simulink model "finalcode"  (R2020a)
settings: Solver=FixedStepDiscrete  StartTime=0.0  StopTime=1  FixedStep=0.0005  RelTol=1e-3  EnableMultiTasking=on
undefined symbols (not defined in the file): acc_calmax1, acc_calmax2, acc_calmin1, acc_calmin2, akemancanshu, angle_middle, bre, bre_calmax, bre_calmin, chasuniujvvvv_hou, chasuniujvvvv_qian, chasuuuu, ecucoder_acal, I_AN01_5K1, I_AN03_5V, I_AN04_5V, kd, kddd, ki, kiii, kp, kppp, leftmax, O_SW06_HS1A, P11111, P22222, PIDmodel, PPPP, rightmax, slip, slip_big, slip_little, slipmodel, T_add, T_del, tiaoshi, TTTTTyouren, vvvv, zhiling
libraries: ec5744lib x305, canmsglib x97, simulink x23
(part 9 of 11)

== matlab function finalcode/转向自动标定/转向自动标定/Subsystem/MATLAB Function ==
  data: steer output; y output; rm input; lm input; bianmaqi input; k output; d output
function [steer,y,k,d] = fcn(rm,lm,bianmaqi)
%使用前请将转向打到最左侧
lm=lm+3000;
rm=rm-3000;
k=0;
d=0;
  persistent i  A B;
     % 初始化状态变量
    if isempty(i)
        i = 0;
        A=zeros(120,1);
        B=zeros(120,1);
    end
 
    if i>20&&i<=140  
        j=i-20;
        delta=(rm-lm)/120;
        steer= lm+j*delta ;
        if (j>=1&&j<=120)
            B(j,1)=steer-delta;
            A(j,1)=bianmaqi;
        end
        
    else
      if i>=140
            N=length(A);
%             bb=0;
%             aa=0;
%             for l=1:120
%                 bbb=bb+B(l,1);
%                 aaa=aa+A(l,1);
%             end
%             bbar=bbb/120;
%             abar=aaa/120;
            k=(sum(B.*A)-N*mean(B)*mean(A))/(sum(A.^2)-N*mean(A)^2);
            d=mean(B)-k*mean(A);
%             steer=single(d);
        end
        steer=lm;
    end

    i=i+1;
  persistent time  a b;
     % 初始化状态变量
    if isempty(time)
        time = 0;
   
        a=5;
        b=10;
    end
    if mod(abs(time), 2) == 0
        result = 1;
    else
        result = 0;
    end
    if time<b&&result==0
    y=6;
 
    elseif time<b&&result==1
    y=15;
  
    elseif time>=b
        if result==1
            y=79;
        else
            y=63;
        end
    else
        y=6;
    end   
    time=time+1;
 
%     
%       persistent time1;
%      % 初始化状态变量
%     if isempty(time1)
%         time1 = 0;
%     end
%     if mod(time1, 2) == 0
%         result1 = 1;
%     else
%         result1 = 0;
%     end
%     if time1<2
%     y=6;
%  
%     elseif time1>=2&&time1<4
%     y=15;
%   
%     elseif time1>=4
%         if result1==1
%             y=79;
%         else
%             y=63;
%         end
%     else
%         y=6;
%     end   
%     time1=time1+1;
   
end

== matlab function finalcode/Subsystem/run/analog_input/有人/踏板标定/踏板冲突 ==
  data: acc_fin_sig1 input; y output; acc_fin_sig2 input; bre_ori_sig input; bre input
function y = fcn(acc_fin_sig1,  acc_fin_sig2,bre_ori_sig,bre)
if (acc_fin_sig1>0.3&&bre_ori_sig+bre>=1)||bre_ori_sig+bre>=2
    y=0;
elseif (acc_fin_sig1==0||acc_fin_sig2==0)
    y=0;
else
    y=acc_fin_sig2;
end

== matlab function finalcode/Subsystem/run/analog_input/有人/踏板标定/Subsystem1/MATLAB Function ==
  data: u input; y output
function y = fcn(u)
if u==0
    y=0;
else
    y=1;
end

== matlab function finalcode/Subsystem/run/analog_input/有人/Subsystem1/MATLAB Function ==
  data: v input; T output
function T = fcn(v)
%#codegen
if v<6000*1.88e-3
    T=2100;
elseif v>11000*1.88e-3
    T=800;
else
    T=1100;
end

== matlab function finalcode/Subsystem/run/analog_input/有人/Subsystem1/MATLAB Function1 ==
  data: T input; TP output
function TP= fcn(T)
if T<10
    TP=0;
else
    TP=T;
end

== matlab function finalcode/Subsystem/run/ctrl/Subsystem1/control_strategy/E,H ==
  data: A input; E output; B input; Q input; R input; F input; N input; H output; J output
function [E,H,J] = MPC_Matrices(A,B,Q,R,F,N)
    n=size(A,1); % A是n*n矩阵,得到n
    p=size(B,2); % B是n*p矩阵,得到p
    M=[eye(n);zeros(N*n,n)]; % 初始化M矩阵,M矩阵是(N+1)n*n的,
                             % 它上面是n*n个"I",这一步先把下半部分写成0
    C=zeros((N+1)*n,N*p); % 初始化C矩阵,这一步令它有(N+1)n*NP个0
     D=zeros(1,N*p);
    % 定义M和C
    tmp=eye(n); % 定义一个n*n 的 I 矩阵
    % 更新Ｍ和C
    for i=1:N % 循环,i从1到N
        rows =i*n+(1:n); %定义当前行数,从i*n开始，共n行
        C(rows,:)=[tmp*B,C(rows-n, 1:end-p)]; %将c矩阵填满
        tmp= A*tmp; %每一次将tmp左乘一次A
        M(rows,:)=tmp; %将M矩阵写满
    end
    % 定义Q_bar和R_bar
    Q_bar = kron(eye(N),Q);
    Q_bar = blkdiag(Q_bar,F);
    R_bar = kron(eye(N),R);
    % 计算G,E,H
    G=M'*Q_bar*M; % G: n*n
    E=C'*Q_bar*M; % E: NP*n
    H=C'*Q_bar*C+R_bar; % NP*NP
for i=1:N % 循环,i从1到N
     D(i)= 0.17;
end
  J=C'*Q_bar*D'

== matlab function finalcode/Subsystem/run/ctrl/Subsystem1/control_strategy/MATLAB Function ==
  data: slip_ratio_fl input; torque_cmd_fl output; slip_ratio_fr input; slip_ratio_rl input; slip_ratio_rr input; desired_slip_ratio input; driver_torque_cmd_fl input; driver_torque_cmd_fr input; driver_torque_cmd_rl input; driver_torque_cmd_rr input; dt input; B input; C input; D input; E input; wheel_radius input; torque_cmd_fr output; torque_cmd_rl output; torque_cmd_rr output
function [torque_cmd_fl, torque_cmd_fr, torque_cmd_rl, torque_cmd_rr] = SlipRatioControlWithMagicFormula(slip_ratio_fl, slip_ratio_fr, slip_ratio_rl, slip_ratio_rr, desired_slip_ratio, driver_torque_cmd_fl, driver_torque_cmd_fr, driver_torque_cmd_rl, driver_torque_cmd_rr, dt, B, C, D, E, wheel_radius)

    % 定义持久变量来存储每个轮胎的上一次误差
    persistent e_prev_fl e_prev_fr e_prev_rl e_prev_rr
    if isempty(e_prev_fl)
        e_prev_fl = 0; e_prev_fr = 0; e_prev_rl = 0; e_prev_rr = 0;
    end

    % 滑膜设计参数
    lambda = 2;            
    K = 0.2;               
    delta = 0.05;          

    % 定义一个内部函数来为每个轮胎进行滑膜控制
    function [torque_cmd, e_prev] = singleWheelControl(slip_ratio, desired_slip_ratio, driver_torque_cmd, e_prev, B, C, D, E, wheel_radius)
        % 计算误差和误差的变化率
        e = desired_slip_ratio - slip_ratio;
        e_dot = (e - e_prev) / dt;
        s = e_dot + lambda * e;

        % 使用Magic Formula计算期望的轮胎纵向力
        Fx_desired = D * sin(C * atan(B * desired_slip_ratio - E*(B * desired_slip_ratio - atan(B * desired_slip_ratio))));
        
        % 转换纵向力为期望扭矩
        desired_torque = Fx_desired * wheel_radius;

        % 根据滑模控制策略调整扭矩
        if abs(s) < delta
            torque_adjustment = 0;
        else
            torque_adjustment = K * s;
        end

        % 结合Magic Formula期望扭矩和滑模控制调整来计算输出扭矩
        torque_cmd = desired_torque + torque_adjustment;
        
        % 保证输出扭矩为非负
        torque_cmd = max(0, torque_cmd); 

        % 更新误差以供下次使用
        e_prev = e;
    end

    % 为每个轮胎应用滑模控制策略
    [torque_cmd_fl, e_prev_fl] = singleWheelControl(slip_ratio_fl, desired_slip_ratio, driver_torque_cmd_fl, e_prev_fl, B, C, D, E, wheel_radius);
    [torque_cmd_fr, e_prev_fr] = singleWheelControl(slip_ratio_fr, desired_slip_ratio, driver_torque_cmd_fr, e_prev_fr, B, C, D, E, wheel_radius);
    [torque_cmd_rl, e_prev_rl] = singleWheelControl(slip_ratio_rl, desired_slip_ratio, driver_torque_cmd_rl, e_prev_rl, B, C, D, E, wheel_radius);
    [torque_cmd_rr, e_prev_rr] = singleWheelControl(slip_ratio_rr, desired_slip_ratio, driver_torque_cmd_rr, e_prev_rr, B, C, D, E, wheel_radius);

end

== matlab function finalcode/Subsystem/run/ctrl/Subsystem1/control_strategy/MATLAB Function1 ==
  data: y output; angle input
function y = fcn(angle)
if angle>30||angle<-30%4650000,4870000,4741002
    y=1;
else
    y = 0;
end

== matlab function finalcode/Subsystem/run/ctrl/Subsystem1/control_strategy/MATLAB Function2 ==
  data: A output; B output; Q output; R output; F output; N output; p output
function [A,B,Q,R,F,N,p] = fcn()
% 定义状态矩阵 A, n*n 矩阵
A = 0;
% 定义输入矩阵 B, n*p 矩阵
R=1;
FN=1;
K=6.89;
B = R/(FN*K);
p = size(B,2);
% 定义Q矩阵，n*n 矩阵
Q = 100;
% 定义F矩阵，n*n 矩阵
F = 100;
% 定义R矩阵，p*p 矩阵
R = 1;
%定义预测区间K
N = 5;

== matlab function finalcode/Subsystem/Tx/TX控制器/速度/188右后/MATLAB Function6 ==
  data: v input; T output; a input
function T = fcn(v,a)
% if a>5
%     y = u;
% elseif a>3&&a<5
%     y=1200;
% else
%     y=800;
% end

if v<6000*1.88e-3
    T=2100;
elseif v>11000*1.88e-3
    T=800;
else
    T=1100;
end

== matlab function finalcode/Subsystem/run/ctrl/Subsystem1/control_strategy/MATLAB Function3 ==
  data: y output; angle input
function y = fcn(angle)
if angle>10||angle<-10%4650000,4870000,4741002
    y=1;
else
    y = 0;
end

== matlab function finalcode/Subsystem/run/ctrl/Subsystem1/control_strategy/MPC ==
  data: X_K input; y output; Prediction input; A input; B input; Q input; R input; F input
function y = fcn(X_K,Prediction,A,B,Q,R,F)
    U_K(:,k) = Prediction;
    % 计算第k+1步时状态变量的值
%     X_K(:,k+1) = (A*X_K(:,k) + B*U_K(:,k))-0.17*A;
end

== matlab function finalcode/Subsystem/run/ctrl/Subsystem1/control_strategy/Subsystem/defuzzification ==
  data: dnb input; delta output; dns input; do input; dps input; dpb input; d1 input; d2 input; d3 input
function delta = fcn(dnb,dns,do,dps,dpb, d1,d2,d3)
delta = dnb*d1/3 + dns*d1 + do*d2 + dps*d3 + dpb*(1-d3/3);
end

== matlab function finalcode/Subsystem/run/ctrl/Subsystem1/control_strategy/Subsystem/α sets ==
  data: alpha input; as output; am output; ab output; a1 input; a2 input
function [as,am,ab] = fcn(alpha, a1, a2)
if alpha < a1
    as = 1-(alpha/a1);
    am = alpha/a1;
    ab = 0;
elseif alpha < a2
    as = 0; 
    am = 1-(alpha-a1)/(a2-a1);
    ab = (alpha-a1)/(a2-a1);
else
    as = 0;
    am = 0;
    ab = 1;
end

== matlab function finalcode/Subsystem/run/ctrl/Subsystem1/control_strategy/Subsystem/β sets ==
  data: beta input; bnb output; bns output; bo output; b1 input; b2 input; bps output; bpb output; b3 input
function [bnb,bns,bo,bps,bpb] = fcn(beta, b1, b2, b3)
if beta < b1
    bnb = 1-(beta+1)/(b1+1);
    bns = (beta+1)/(b1+1);
    bo  = 0;
    bps = 0;
    bpb = 0;
elseif beta < b2
    bnb = 0; 
    bns = 1-(beta-b1)/(b2-b1);
    bo = (beta-b1)/(b2-b1);
    bps = 0;
    bpb = 0;
elseif beta < b3
    bnb = 0;
    bns = 0;
    bo  = 1-(beta-b2)/(b3-b2);
    bps = (beta-b2)/(b3-b2);
    bpb = 0;
else
    bnb = 0;
    bns = 0;
    bo  = 0;
    bps = 1-(beta-b3)/(1-b3);
    bpb = (beta-b3)/(1-b3);
end

== matlab function finalcode/Subsystem/run/ctrl/Subsystem1/control_strategy/差速/MATLAB Function3 ==
  data: u input; youhou output; M input; youqian output; zuohou output; zuoqian output
function [youhou,youqian,zuohou,zuoqian] = fcn(u,M)
% U=4*u;
r=0.2032;%轮半径
B1=1.18;%左右轮距
B2=1.16;
youqian=M*r/(2*B2)+u;
youhou=youqian;
zuoqian=-M*r/(2*B1)+u;
zuohou=zuoqian;
end

== matlab function finalcode/Subsystem/run/ctrl/Subsystem1/control_strategy/差速/差速/LQR差速 ==
  data: yaw_error input; M output; yaw_rate input; J input
% function M = carLQRControl(yaw_error, yaw_rate,J)
%     % 赛车LQR控制器参数
%     Q = diag([1, 1]); % 状态误差权重矩阵
%     R = 0.1; % 控制输入权重
%     
%     % 定义车辆模型参数
%     % J转动惯量
%     
%     % 设计LQR增益矩阵 K
%     A = [0, 1; 0, 0];%输入为期望与实际横摆力矩差值和横摆角速度
%     B = [0; J];
%     K = lqr(A, B, Q, R);
%     
%     % 计算横摆力矩控制输入
%     M = -K* [yaw_error; yaw_rate];
function M = carLQRControl(yaw_error, yaw_rate,J)
    % 赛车LQR控制器参数
    Q = diag([1, 1]); % 状态误差权重矩阵
    R = 0.1; % 控制输入权重
    
    % 设计LQR增益矩阵 K
    A = [0, 1; 0, 0]; % 输入为期望与实际横摆力矩差值和横摆角速度
    B = [0; J];
    
    % 使用迭代法求解代数Riccati方程，计算LQR增益矩阵 K
    max_iterations = 20;
    tolerance = 1e-2;
    P = eye(size(A));
%     for i = 1:max_iterations
%         P_new = Q + A' * P * A - A' * P * B * (R + B' * P * B)^(-1) * B' * P * A;
%         if max(abs(P_new - P), [], 'all') < tolerance
%             P = P_new;
%             break;
%         end
%         P = P_new;
%   K = (R + B' * P * B)^(-1) * B' * P * A;
%     end
     % 计算LQR增益矩阵 

 
   for k = 1:max_iterations
        F = inv(R+B'*P*B)*B'*P*A;
        P_new = (A-B*F)'*P*(A-B*F)+(F)'*R*(F)+Q;
        if max(abs(P_new - P), [], 'all') < tolerance
             P= P_new;
             F = inv(R+B'*P*B)*B'*P*A;
            break;
        end
        P= P_new;
    end
    F_N=F; 
   
    % 计算横摆力矩控制输入
    M = -F_N * [yaw_error; yaw_rate];

end

== matlab function finalcode/Subsystem/Tx/TX控制器/速度/189左后/MATLAB Function2 ==
  data: enable input; enable_1 input; T input; TargetVelocity output; AMK_TorqueLimitPositive output; enable output; errorreset output; blnverteron output; CAN_dbcon output; v input
function [TargetVelocity,AMK_TorqueLimitPositive,enable,errorreset,blnverteron,CAN_dbcon]= fcn(enable,enable_1,T,v)
if (enable_1==0)
    TargetVelocity=0;
    enable=0;
    errorreset=1;
    blnverteron=0;
    CAN_dbcon=0;
    AMK_TorqueLimitPositive=0;
elseif (enable==0 && enable_1==1)
    TargetVelocity=2000;
    enable=1;
    errorreset=0;
    blnverteron=1;
    CAN_dbcon=1;
    AMK_TorqueLimitPositive=0;
elseif (enable==1 && enable_1==1)
    TargetVelocity=2000;
    enable=1;
    errorreset=0;
    blnverteron=1;
    CAN_dbcon=1;
    AMK_TorqueLimitPositive=T;
else
    TargetVelocity=0;
    enable=0;
    errorreset=1;
    blnverteron=0;
    CAN_dbcon=0;
    AMK_TorqueLimitPositive=0;
end

end

== matlab function finalcode/Subsystem/run/ctrl/Subsystem1/control_strategy/差速/差速/MATLAB Function ==
  data: u input; y output
function y = fcn(u)

y = u;

== matlab function finalcode/Subsystem/run/ctrl/Subsystem1/control_strategy/差速/差速/pid ==
  data: v input; u input; v_zuoqian output
function v_zuoqian  = carPIDControl(v, u)
    % 赛车PID控制器参数
    kp = 0.2;
    ki = 0.1;
    kd = 0.01;
    
    % 状态变量
    persistent integral previous_error 
    
    % 初始化状态变量
    if isempty(integral)
        integral = 0;
        previous_error = 0;
        i=0;
    end
    
    % PID控制器计算
    error = u - v;
    integral = integral + error*0.02;
    derivative = (error - previous_error)/0.02;
    
        if integral > 0.4    
        integral = 0.4;
        end
        if integral < -0.4    
        integral = -0.4;
        end
    
   v_zuoqian = kp * error + ki * integral + kd * derivative;
   
    % 保存上一个误差用于下次计算
    previous_error = error;
end

== matlab function finalcode/Subsystem/run/ctrl/Subsystem1/control_strategy/差速/差速/pid1 ==
  data: v input; u input; v_zuoqian output
function v_zuoqian  = carPIDControl(v, u)
    % 赛车PID控制器参数
    kp = 0.2;
    ki = 0.1;
    kd = 0.01;
    
    % 状态变量
    persistent integral previous_error 
    
    % 初始化状态变量
    if isempty(integral)
        integral = 0;
        previous_error = 0;
        i=0;
    end
    
    % PID控制器计算
    error = u - v;
    integral = integral + error*0.02;
    derivative = (error - previous_error)/0.02;
    
        if integral > 0.4    
        integral = 0.4;
        end
        if integral < -0.4    
        integral = -0.4;
        end
    
   v_zuoqian = kp * error + ki * integral + kd * derivative;
   
    % 保存上一个误差用于下次计算
    previous_error = error;
end

== matlab function finalcode/Subsystem/run/ctrl/Subsystem1/control_strategy/差速/差速/pid2 ==
  data: v input; u input; v_zuoqian output
function v_zuoqian  = carPIDControl(v, u)
    % 赛车PID控制器参数
    kp = 0.2;
    ki = 0.1;
    kd = 0.01;
    
    % 状态变量
    persistent integral previous_error 
    
    % 初始化状态变量
    if isempty(integral)
        integral = 0;
        previous_error = 0;
        i=0;
    end
    
    % PID控制器计算
    error = u - v;
    integral = integral + error*0.02;
    derivative = (error - previous_error)/0.02;
    
        if integral > 0.4    
        integral = 0.4;
        end
        if integral < -0.4    
        integral = -0.4;
        end
    
   v_zuoqian = kp * error + ki * integral + kd * derivative;
   
    % 保存上一个误差用于下次计算
    previous_error = error;
end

== matlab function finalcode/Subsystem/run/ctrl/Subsystem1/control_strategy/差速/差速/pid3 ==
  data: v input; u input; v_zuoqian output
function v_zuoqian  = carPIDControl(v, u)
    % 赛车PID控制器参数
    kp = 0.2;
    ki = 0.1;
    kd = 0.01;
    
    % 状态变量
    persistent integral previous_error 
    
    % 初始化状态变量
    if isempty(integral)
        integral = 0;
        previous_error = 0;
        i=0;
    end
    
    % PID控制器计算
    error = u - v;
    integral = integral + error*0.02;
    derivative = (error - previous_error)/0.02;
    
        if integral > 0.4    
        integral = 0.4;
        end
        if integral < -0.4    
        integral = -0.4;
        end
    
   v_zuoqian = kp * error + ki * integral + kd * derivative;
   
    % 保存上一个误差用于下次计算
    previous_error = error;
end

== matlab function finalcode/Subsystem/run/ctrl/Subsystem1/control_strategy/差速/差速/期望横摆力矩计算 ==
  data: delta input; Mz output; Vx input; ax input
function Mz = calculateYawMoment(delta,  Vx, ax)
    % 输入参数：
    % delta: 前轮转角 (rad)
    % Vx: 车辆速度 (m/s)
    % ax: 侧向加速度 (m/s^2)
    m=210;%: 车辆质量 (kg)
     lf=0.765;%: 前轴到重心的距离 (m)
     lr=0.765;%: 后轴到重心的距离 (m)
    
    % 轮胎侧向力估计，这里使用一个简化的线性模型
    Fy = ax * (lr * m * 9.81) / (lf + lr);
    delta=delta*pi/180
    % 计算期望的横摆力矩
    Mz = lf * Fy * cos(delta);
end

== matlab function finalcode/Subsystem/run/ctrl/Subsystem1/control_strategy/差速/差速/阿克曼转向 ==
  data: wfl output; v input; wfr output; wrl output; wrr output; a input; angle input
function [wfl,wfr,wrl,wrr]= fcn(v,a,angle)
%22e轴距：1170mm 轮距 1530mm 前47%后53%即，前0.72后0.81 
L=1.53;%前后轴距    u是转角
d=1.17;%车宽
c1=0.93;%前车对角线的一半
c2=1;
k=1;%12.641传动比

Rcg=v^2/a;
if angle<0
    Rfr=sqrt(c1^2+Rcg^2-2*c1*Rcg*cos(2.25));
    Rfl=sqrt(c1^2+Rcg^2-2*c1*Rcg*cos(0.89));
    Rrl=sqrt(c2^2+Rcg^2-2*c2*Rcg*cos(0.945));
    Rrr=sqrt(c2^2+Rcg^2-2*c2*Rcg*cos(2.2));
    wfl=k*v/Rcg*Rfl;
    wfr=k*v/Rcg*Rfr;
    wrl=k*v/Rcg*Rrl;
    wrr=k*v/Rcg*Rrr;
else
    Rfl=sqrt(c1^2+Rcg^2-2*c1*Rcg*cos(2.25));
    Rfr=sqrt(c1^2+Rcg^2-2*c1*Rcg*cos(0.89));
    Rrr=sqrt(c2^2+Rcg^2-2*c2*Rcg*cos(0.945));
    Rrl=sqrt(c2^2+Rcg^2-2*c2*Rcg*cos(2.2));
    wfl=k*v/Rcg*Rfl;
    wfr=k*v/Rcg*Rfr;
    wrl=k*v/Rcg*Rrl;
    wrr=k*v/Rcg*Rrr; 
end
wfl=594.06*min(wfl,v+2);
wfr=594.06*min(wfr,v+2);
wrl=594.06*min(wrl,v+2);
wrr=594.06*min(wrr,v+2);
wfl=594.06*max(wfl,v-2);
wfr=594.06*max(wfr,v-2);
wrl=594.06*max(wrl,v-2);
wrr=594.06*max(wrr,v-2);

== matlab function finalcode/Subsystem/run/ctrl/Subsystem1/control_strategy/滑模控制 ==
  data: slip_ratio_fl input; slip_ratio_fr input; slip_ratio_rl input; slip_ratio_rr input; torque_cmd_fl output; driver_torque_cmd_fl input; driver_torque_cmd_fr input; driver_torque_cmd_rl input; driver_torque_cmd_rr input; torque_cmd_fr output; torque_cmd_rl output; torque_cmd_rr output
function [torque_cmd_fl, torque_cmd_fr, torque_cmd_rl, torque_cmd_rr] = SlipRatioControl(slip_ratio_fl, slip_ratio_fr, slip_ratio_rl, slip_ratio_rr,   driver_torque_cmd_fl, driver_torque_cmd_fr, driver_torque_cmd_rl, driver_torque_cmd_rr)

    % 每个轮都有自己的误差历史记录
    persistent e_prev_fl e_prev_fr e_prev_rl e_prev_rr i driver_weight
    if isempty(e_prev_fl)
        e_prev_fl = 0; e_prev_fr = 0; e_prev_rl = 0; e_prev_rr = 0;
        driver_weight = 0.5;  % 车手命令的权重
        i=0;
    end

    % 设定参数
    lambda = 3;            % 滑模面设计参数
    K = 0.5;               % 滑模增益
    delta = 0.05;          % 滑模边界，小于此值时不做扭矩调整
%     driver_weight = 0.05;  % 车手命令的权重
    desired_slip_ratio=0.2;
    % 定义一个内部函数来进行滑膜控制，这样可以为每个轮重复使用
    function [torque_cmd, e_prev,e] = singleWheelControl(slip_ratio, desired_slip_ratio, driver_torque_cmd, e_prev)
        % 计算误差和误差的变化率
        e = desired_slip_ratio - slip_ratio;
        e_dot = (e - e_prev) / 0.02;
        s = e_dot + lambda * e;

        % 滑模控制策略
        if abs(s) < delta
            torque_adjustment = 0;  % s小于滑模边界时不做调整
        else
            torque_adjustment = K * s;  % 根据s的符号进行扭矩调整
        end

        % 结合车手的扭矩命令，并应用滑模控制的调整
        torque_cmd = driver_torque_cmd + driver_weight * driver_torque_cmd * torque_adjustment;
        torque_cmd = max(0, torque_cmd);  % 保证扭矩命令为正
        torque_cmd = min(2000, torque_cmd);  % 保证扭矩小于2000

        % 更新误差
        e_prev = e;
    end
    % 对每个轮应用滑模控制策略
    [torque_cmd_fl, e_prev_fl,efl] = singleWheelControl(slip_ratio_fl, desired_slip_ratio, driver_torque_cmd_fl, e_prev_fl);
    [torque_cmd_fr, e_prev_fr,efr] = singleWheelControl(slip_ratio_fr, desired_slip_ratio, driver_torque_cmd_fr, e_prev_fr);
    [torque_cmd_rl, e_prev_rl,erl] = singleWheelControl(slip_ratio_rl, desired_slip_ratio, driver_torque_cmd_rl, e_prev_rl);
    [torque_cmd_rr, e_prev_rr,err] = singleWheelControl(slip_ratio_rr, desired_slip_ratio, driver_torque_cmd_rr, e_prev_rr);
     %安全程序
     if (efl>0.8||efr>0.8||erl>0.8||err>0.8)
         i=i+1;
         if i>100
             driver_weight=0;
         end
     end
     if (efl<0.3&&efr<0.3&&erl<0.3&&err<0.3)
         i=0;
     end

end

== matlab function finalcode/Subsystem/run/ctrl/Subsystem1/control_strategy/限滑/MATLAB Function ==
  data: slip_ratio_front_left input; torque_front_left output; slip_ratio_front_right input; slip_ratio_rear_left input; slip_ratio_rear_right input; e_prev input; dt input; torque_front_right output; torque_rear_left output; torque_rear_right output
function [torque_front_left, torque_front_right, torque_rear_left, torque_rear_right] = SlipRatioControl(slip_ratio_front_left, slip_ratio_front_right, slip_ratio_rear_left, slip_ratio_rear_right,  e_prev, dt)

% 参数设定
lambda = 5; % 调整因子，用于滑模面设计，实际应用中可能需要调整
boundary_thickness = 0.1; % 边界层厚度，用于sigmoid函数，以确保输出在合理范围内
max_torque = 2000; % 最大扭矩，表示车辆能够输出的最大扭矩
slip_ratio_desired=0.2;
% 内部函数，为每个轮子计算扭矩
function torque = computeTorque(slip_ratio_actual, e_prev)
    % 计算误差及其导数
    e = slip_ratio_desired - slip_ratio_actual;
    e_dot = (e - e_prev) / dt;
    
    % 滑模控制
    s = e_dot + lambda * e;
    
    % 使用软饱和函数（sigmoid函数）计算扭矩指令
    torque = max_torque / (1 + exp(-10 * (s - boundary_thickness)));
    
    % 限制扭矩值
    torque = min(max_torque, torque);
end

% 为每个轮子计算扭矩
torque_front_left = computeTorque(slip_ratio_front_left, e_prev(1));
torque_front_right = computeTorque(slip_ratio_front_right, e_prev(2));
torque_rear_left = computeTorque(slip_ratio_rear_left, e_prev(3));
torque_rear_right = computeTorque(slip_ratio_rear_right, e_prev(4));

% 更新上一次的误差
e_prev(1) = slip_ratio_desired - slip_ratio_front_left;
e_prev(2) = slip_ratio_desired - slip_ratio_front_right;
e_prev(3) = slip_ratio_desired - slip_ratio_rear_left;
e_prev(4) = slip_ratio_desired - slip_ratio_rear_right;

end

== matlab function finalcode/Subsystem/run/ctrl/Subsystem1/control_strategy/限滑/MPC/MPC/MATLAB Function ==
  data: u input; y output
function y = fcn(u)
if u>=0.169&&u<=0.17
    y=1;
else
    y=0;
end

end

== matlab function finalcode/Subsystem/run/ctrl/Subsystem1/control_strategy/限滑/MPC/MPC/MATLAB Function1 ==
  data: u input; y output
function y = fcn(u)
if u>=0.169&&u<=0.17
    y=1;
else
    y=0;
end

end

== matlab function finalcode/Subsystem/run/ctrl/Subsystem1/control_strategy/限滑/MPC/MPC/MATLAB Function2 ==
  data: u input; y output
function y = fcn(u)

if u>=0.169&&u<=0.17
    y=1;
else
    y=0;
end

end

== matlab function finalcode/Subsystem/run/ctrl/Subsystem1/control_strategy/限滑/MPC/MPC/MATLAB Function3 ==
  data: u input; y output
function y = fcn(u)

if u>=0.169&&u<=0.17
    y=1;
else
    y=0;
end

end

== matlab function finalcode/Subsystem/run/ctrl/Subsystem1/control_strategy/限滑/MPC/MPC/MPC右前/MPC_function ==
  data: x_k input; u_k output; U_init input
function u_k= Prediction(x_k,U_init)
% 定义状态矩阵 A, n*n 矩阵
A = 0;
% 定义输入矩阵 B, n*p 矩阵
R=0.2032;
FN=2058;
K=6.89;
B = R/(FN*K);
p = size(B,2);
% 定义Q矩阵，n*n 矩阵
Q = 100;
% 定义F矩阵，n*n 矩阵
F = 100;
% 定义R矩阵，p*p 矩阵
R = 1;
% 定义迭代次数和学习率
maxIterations = 5;
learningRate = 0.3;
N=5;%预测区间
n=size(A,1); % A是n*n矩阵,得到n
p=size(B,2); % B是n*p矩阵,得到p
M=[eye(n);zeros(N*n,n)]; % 初始化M矩阵,M矩阵是(N+1)n*n的
D=[0.17;zeros(N*n,n)];
C=zeros((N+1)*n,N*p); % 初始化C矩阵,这一步令它有(N+1)n*NP个0

% 定义M和C
tmp=eye(n); % 定义一个n*n 的 I 矩阵
    for i=1:N % 循环,i从1到N
        rows =i*n+(1:n); %定义当前行数,从i*n开始，共n行
        C(rows,:)=[tmp*B,C(rows-n, 1:end-p)]; %将c矩阵填满
        tmp= A*tmp; %每一次将tmp左乘一次A
        M(rows,:)=tmp; %将M矩阵写满
         D(rows,:)=0.17;
    end
    % 定义Q_bar和R_bar
    Q_bar = kron(eye(N),Q);
    Q_bar = blkdiag(Q_bar,F);
    R_bar = kron(eye(N),R);
    % 计算G,E,H
    G=M'*Q_bar*M; % G: n*n
    E=C'*Q_bar*M; % E: NP*n
    H=C'*Q_bar*C+R_bar; % NP*NP
 J=(D'*Q_bar*C)';
 L=E*x_k+J;
 U = U_init*ones(N*p,1); % NP x 1
%  options = optimoptions('quadprog', 'Algorithm', 'active-set');
%  U_k = quadprog(H,L, [], [], [], [], 0*ones(5,1), 1100*ones(5,1), 100*ones(5,1), options);
    % 梯度下降法求解最优二次规划问题
    G=size(U,1);
    S=zeros(G*maxIterations,1);
    for i = 1:maxIterations
        % 计算目标函数的梯度
        gradient = 2*H*U + 2*L;
        % 更新变量 U，并保持在 [0, 1100] 范围内
        U = U - learningRate * gradient;
        U = max(U, 0);
        U = min(U, 1100);
        O=(i-1)*maxIterations+(1:maxIterations);
        S(O,1)=U;
    end

 u_k = S(1:p,1); % 取第一个结果
end

== matlab function finalcode/Subsystem/run/ctrl/Subsystem1/control_strategy/限滑/MPC/MPC/MPC右后/MPC_function ==
  data: x_k input; u_k output; U_init input
function u_k= Prediction(x_k,U_init)
% 定义状态矩阵 A, n*n 矩阵
A = 0;
% 定义输入矩阵 B, n*p 矩阵
R=0.2032;
FN=2058;
K=6.89;
B = R/(FN*K);
p = size(B,2);
% 定义Q矩阵，n*n 矩阵
Q = 100;
% 定义F矩阵，n*n 矩阵
F = 100;
% 定义R矩阵，p*p 矩阵
R = 1;
% 定义迭代次数和学习率
maxIterations = 5;
learningRate = 0.3;
N=5;%预测区间
n=size(A,1); % A是n*n矩阵,得到n
p=size(B,2); % B是n*p矩阵,得到p
M=[eye(n);zeros(N*n,n)]; % 初始化M矩阵,M矩阵是(N+1)n*n的
D=[0.17;zeros(N*n,n)];
C=zeros((N+1)*n,N*p); % 初始化C矩阵,这一步令它有(N+1)n*NP个0

% 定义M和C
tmp=eye(n); % 定义一个n*n 的 I 矩阵
    for i=1:N % 循环,i从1到N
        rows =i*n+(1:n); %定义当前行数,从i*n开始，共n行
        C(rows,:)=[tmp*B,C(rows-n, 1:end-p)]; %将c矩阵填满
        tmp= A*tmp; %每一次将tmp左乘一次A
        M(rows,:)=tmp; %将M矩阵写满
         D(rows,:)=0.17;
    end
    % 定义Q_bar和R_bar
    Q_bar = kron(eye(N),Q);
    Q_bar = blkdiag(Q_bar,F);
    R_bar = kron(eye(N),R);
    % 计算G,E,H
    G=M'*Q_bar*M; % G: n*n
    E=C'*Q_bar*M; % E: NP*n
    H=C'*Q_bar*C+R_bar; % NP*NP
 J=(D'*Q_bar*C)';
 L=E*x_k+J;
 U = U_init*ones(N*p,1); % NP x 1
%  options = optimoptions('quadprog', 'Algorithm', 'active-set');
%  U_k = quadprog(H,L, [], [], [], [], 0*ones(5,1), 1100*ones(5,1), 100*ones(5,1), options);
    % 梯度下降法求解最优二次规划问题
    G=size(U,1);
    S=zeros(G*maxIterations,1);
    for i = 1:maxIterations
        % 计算目标函数的梯度
        gradient = 2*H*U + 2*L;
        % 更新变量 U，并保持在 [0, 1100] 范围内
        U = U - learningRate * gradient;
        U = max(U, 0);
        U = min(U, 1100);
        O=(i-1)*maxIterations+(1:maxIterations);
        S(O,1)=U;
    end

 u_k = S(1:p,1); % 取第一个结果
end

== matlab function finalcode/Subsystem/run/ctrl/Subsystem1/control_strategy/限滑/MPC/MPC/MPC左前/MPC_function ==
  data: x_k input; u_k output; U_init input
function u_k= Prediction(x_k,U_init)
% 定义状态矩阵 A, n*n 矩阵
A = 0;
% 定义输入矩阵 B, n*p 矩阵
R=0.2032;
FN=2058;
K=6.89;
B = R/(FN*K);
p = size(B,2);
% 定义Q矩阵，n*n 矩阵
Q = 100;
% 定义F矩阵，n*n 矩阵
F = 100;
% 定义R矩阵，p*p 矩阵
R = 1;
% 定义迭代次数和学习率
maxIterations = 5;
learningRate = 0.3;
N=5;%预测区间
n=size(A,1); % A是n*n矩阵,得到n
p=size(B,2); % B是n*p矩阵,得到p
M=[eye(n);zeros(N*n,n)]; % 初始化M矩阵,M矩阵是(N+1)n*n的
D=[0.17;zeros(N*n,n)];
C=zeros((N+1)*n,N*p); % 初始化C矩阵,这一步令它有(N+1)n*NP个0

% 定义M和C
tmp=eye(n); % 定义一个n*n 的 I 矩阵
    for i=1:N % 循环,i从1到N
        rows =i*n+(1:n); %定义当前行数,从i*n开始，共n行
        C(rows,:)=[tmp*B,C(rows-n, 1:end-p)]; %将c矩阵填满
        tmp= A*tmp; %每一次将tmp左乘一次A
        M(rows,:)=tmp; %将M矩阵写满
         D(rows,:)=0.17;
    end
    % 定义Q_bar和R_bar
    Q_bar = kron(eye(N),Q);
    Q_bar = blkdiag(Q_bar,F);
    R_bar = kron(eye(N),R);
    % 计算G,E,H
    G=M'*Q_bar*M; % G: n*n
    E=C'*Q_bar*M; % E: NP*n
    H=C'*Q_bar*C+R_bar; % NP*NP
 J=(D'*Q_bar*C)';
 L=E*x_k+J;
 U = U_init*ones(N*p,1); % NP x 1
%  options = optimoptions('quadprog', 'Algorithm', 'active-set');
%  U_k = quadprog(H,L, [], [], [], [], 0*ones(5,1), 1100*ones(5,1), 100*ones(5,1), options);
    % 梯度下降法求解最优二次规划问题
    G=size(U,1);
    S=zeros(G*maxIterations,1);
    for i = 1:maxIterations
        % 计算目标函数的梯度
        gradient = 2*H*U + 2*L;
        % 更新变量 U，并保持在 [0, 1100] 范围内
        U = U - learningRate * gradient;
        U = max(U, 0);
        U = min(U, 1100);
        O=(i-1)*maxIterations+(1:maxIterations);
        S(O,1)=U;
    end

 u_k = S(1:p,1); % 取第一个结果
end

== matlab function finalcode/Subsystem/Tx/TX控制器/速度/189左后/MATLAB Function4 ==
  data: u input; y output; zhidongesc input; zhidongebs input; huanting input
function y = fcn(u,zhidongesc,zhidongebs,huanting)
 y = u*594.06;
if zhidongesc>1800&&zhidongebs==2
    y = u*594.06;
end
if zhidongesc<1500&&zhidongebs==2
    y=0;
end
if huanting~=0
    y=0;
end

== matlab function finalcode/Subsystem/run/ctrl/Subsystem1/control_strategy/限滑/MPC/MPC/MPC左后/MPC_function ==
  data: x_k input; u_k output; U_init input
function u_k= Prediction(x_k,U_init)
% 定义状态矩阵 A, n*n 矩阵
A = 0;
% 定义输入矩阵 B, n*p 矩阵
R=0.2032;
FN=2058;
K=6.89;
B = R/(FN*K);
p = size(B,2);
% 定义Q矩阵，n*n 矩阵
Q = 100;
% 定义F矩阵，n*n 矩阵
F = 100;
% 定义R矩阵，p*p 矩阵
R = 1;
% 定义迭代次数和学习率
maxIterations = 5;
learningRate = 0.3;
N=5;%预测区间
n=size(A,1); % A是n*n矩阵,得到n
p=size(B,2); % B是n*p矩阵,得到p
M=[eye(n);zeros(N*n,n)]; % 初始化M矩阵,M矩阵是(N+1)n*n的
D=[0.17;zeros(N*n,n)];
C=zeros((N+1)*n,N*p); % 初始化C矩阵,这一步令它有(N+1)n*NP个0

% 定义M和C
tmp=eye(n); % 定义一个n*n 的 I 矩阵
    for i=1:N % 循环,i从1到N
        rows =i*n+(1:n); %定义当前行数,从i*n开始，共n行
        C(rows,:)=[tmp*B,C(rows-n, 1:end-p)]; %将c矩阵填满
        tmp= A*tmp; %每一次将tmp左乘一次A
        M(rows,:)=tmp; %将M矩阵写满
         D(rows,:)=0.17;
    end
    % 定义Q_bar和R_bar
    Q_bar = kron(eye(N),Q);
    Q_bar = blkdiag(Q_bar,F);
    R_bar = kron(eye(N),R);
    % 计算G,E,H
    G=M'*Q_bar*M; % G: n*n
    E=C'*Q_bar*M; % E: NP*n
    H=C'*Q_bar*C+R_bar; % NP*NP
 J=(D'*Q_bar*C)';
 L=E*x_k+J;
 U = U_init*ones(N*p,1); % NP x 1
%  options = optimoptions('quadprog', 'Algorithm', 'active-set');
%  U_k = quadprog(H,L, [], [], [], [], 0*ones(5,1), 1100*ones(5,1), 100*ones(5,1), options);
    % 梯度下降法求解最优二次规划问题
    G=size(U,1);
    S=zeros(G*maxIterations,1);
    for i = 1:maxIterations
        % 计算目标函数的梯度
        gradient = 2*H*U + 2*L;
        % 更新变量 U，并保持在 [0, 1100] 范围内
        U = U - learningRate * gradient;
        U = max(U, 0);
        U = min(U, 1100);
        O=(i-1)*maxIterations+(1:maxIterations);
        S(O,1)=U;
    end

 u_k = S(1:p,1); % 取第一个结果
end

== matlab function finalcode/Subsystem/run/ctrl/Subsystem1/control_strategy/限滑/PID限滑/pid限滑与ABS ==
  data: slip input; throttle output; slip_ratio_limit input; brake output; u input
function [throttle, brake] = carPIDWithSlipControl(slip, slip_ratio_limit,u)
    % 赛车PID控制器参数
    kp = 0.2;
    ki = 0.1;
    kd = 0.01;
    
    % 状态变量
    persistent integral previous_error i
    
    % 初始化状态变量
    if isempty(integral)
        integral = 0;
        previous_error = 0;
        i=0;
    end
    
    % PID控制器计算
    error = 0.2 - slip;
    integral = integral + error*0.02;
    derivative = (error - previous_error)/0.02;
    
   k = kp * error + ki * integral + kd * derivative;
    if i<100
    
        output = u+k*u;
        if output>2000
            output=2000;
        end
    else
        output=u;
    end
    % 根据滑移率限制输出
  
    if slip > slip_ratio_limit
        brake = 0;%output;
        throttle = 0;
    else
        brake = 0;
        throttle = output;
    end
    
    % 保存上一个误差用于下次计算
    previous_error = error;

    i=i+1;
end

== matlab function finalcode/Subsystem/run/ctrl/Subsystem1/control_strategy/限滑/PID限滑/pid限滑与ABS1 ==
  data: slip input; throttle output; slip_ratio_limit input; brake output; u input
function [throttle, brake] = carPIDWithSlipControl(slip, slip_ratio_limit,u)
    % 赛车PID控制器参数
    kp = 0.2;
    ki = 0.1;
    kd = 0.01;
    
    % 状态变量
    persistent integral previous_error i
    
    % 初始化状态变量
    if isempty(integral)
        integral = 0;
        previous_error = 0;
        i=0;
    end
    
    % PID控制器计算
    error = 0.2 - slip;
    integral = integral + error*0.02;
    derivative = (error - previous_error)/0.02;
    
   k = kp * error + ki * integral + kd * derivative;
    if i<100
    
        output = u+k*u;
        if output>2000
            output=2000;
        end
    else
        output=u;
    end
    % 根据滑移率限制输出
  
    if slip > slip_ratio_limit
        brake = 0;%output;
        throttle = 0;
    else
        brake = 0;
        throttle = output;
    end
    
    % 保存上一个误差用于下次计算
    previous_error = error;
    i=i+1;
end

== matlab function finalcode/Subsystem/run/ctrl/Subsystem1/control_strategy/限滑/PID限滑/pid限滑与ABS2 ==
  data: slip input; throttle output; slip_ratio_limit input; brake output; u input
function [throttle, brake] = carPIDWithSlipControl(slip, slip_ratio_limit,u)
    % 赛车PID控制器参数
    kp = 0.2;
    ki = 0.1;
    kd = 0.01;
    
    % 状态变量
    persistent integral previous_error i
    
    % 初始化状态变量
    if isempty(integral)
        integral = 0;
        previous_error = 0;
        i=0;
    end
    
    % PID控制器计算
    error = 0.2 - slip;
    integral = integral + error*0.02;
    derivative = (error - previous_error)/0.02;
   k = kp * error + ki * integral + kd * derivative;
    if i<100
    
        output = u+k*u;
        if output>2000
            output=2000;
        end
    else
        output=u;
    end
    % 根据滑移率限制输出
  
    if slip > slip_ratio_limit
        brake = 0;%output;
        throttle = 0;
    else
        brake = 0;
        throttle = output;
    end
    
    % 保存上一个误差用于下次计算
    previous_error = error;
    i=i+1;
end

== matlab function finalcode/Subsystem/run/ctrl/Subsystem1/control_strategy/限滑/PID限滑/pid限滑与ABS3 ==
  data: slip input; throttle output; slip_ratio_limit input; brake output; u input
function [throttle, brake] = carPIDWithSlipControl(slip, slip_ratio_limit,u)
    % 赛车PID控制器参数
    kp = 0.2;
    ki = 0.1;
    kd = 0.01;
    
    % 状态变量
    persistent integral previous_error i
    
    % 初始化状态变量
    if isempty(integral)
        integral = 0;
        previous_error = 0;
        i=0;
    end
    
    % PID控制器计算
    error = 0.2 - slip;
    integral = integral + error*0.02;
    derivative = (error - previous_error)/0.02;
    
   k = kp * error + ki * integral + kd * derivative;
    if i<100
    
        output = u+k*u;
        if output>2000
            output=2000;
        end
    else
        output=u;
    end
    % 根据滑移率限制输出
  
    if slip > slip_ratio_limit
        brake =0;% output;
        throttle = 0;
    else
        brake = 0;
        throttle = output;
    end
    
    % 保存上一个误差用于下次计算
    previous_error = error;
    i=i+1;
end

== matlab function finalcode/Subsystem/run/ctrl/Subsystem1/control_strategy/限滑/PID限滑/计算油压 ==
  data: y1 input; p1 output; y2 input; y3 input; y4 input; p2 output; p3 output; p4 output
function [p1,p2,p3,p4]= fcn(y1,y2,y3,y4)
S=0.000491;
%p1 p2 p3 p4分别是左前、右前、左后、右后油压
p1=y1/(0.8*S)/1000;
p2=y2/(0.8*S)/1000;
p3=y3/(0.4*S)/1000;
p4=y4/(0.4*S)/1000;
% if p1<0
%     p1=0;
%     end
% if p2<0
%     p2=0;
%     end
% if p3<0
%     p3=0;
%     end
% if p4<0
%     p4=0;
% end

== matlab function finalcode/Subsystem/run/ctrl/Subsystem1/control_strategy/限滑/Subsystem1/MATLAB Function2 ==
  data: u input; y output; mpc input; pid input; slip input; model input
function y = fcn(u,mpc,pid,slip,model)
if slip>0.8&&model~=6
    y=pid;
elseif slip>0.165&&slip<0.17
        y=mpc;
else
        y=u;
end
end

== matlab function finalcode/Subsystem/run/ctrl/Subsystem1/control_strategy/限滑/Subsystem1/MATLAB Function3 ==
  data: u input; y output; mpc input; pid input; slip input; model input
function y = fcn(u,mpc,pid,slip,model)
if slip>0.8&&model~=6
    y=pid;
elseif slip>0.169&&slip<0.17
        y=mpc;
else
        y=u;
end
end

== matlab function finalcode/Subsystem/run/ctrl/Subsystem1/control_strategy/限滑/Subsystem1/MATLAB Function4 ==
  data: u input; y output; mpc input; pid input; slip input; model input
function y = fcn(u,mpc,pid,slip,model)
if slip>0.8&&model~=6
    y=pid;
elseif slip>0.165&&slip<0.17
        y=mpc;
else
        y=u;
end
end

== matlab function finalcode/Subsystem/run/ctrl/Subsystem1/control_strategy/限滑/Subsystem1/MATLAB Function5 ==
  data: u input; y output; mpc input; pid input; slip input; model input
function y = fcn(u,mpc,pid,slip,model)
if slip>0.8&&model~=6
    y=pid;
elseif slip>0.165&&slip<0.17
        y=mpc;
else
        y=u;
end
end

== matlab function finalcode/Subsystem/Tx/TX控制器/速度/189左后/MATLAB Function5 ==
  data: v input; y output; angle input; vz input; model input
function y = fcn(v, angle, vz,model)
if(angle>3||angle<-3)&&model==3%4650000,4870000,4741002
    y=vz*594.06;
else
    y = v;
end

== matlab function finalcode/Subsystem/run/滑移率计算 ==
  data: vyouhou input; slipyuohou output; vyouqian input; vzouhou input; vzuoqian input; v input; slipyouqian output; slipzuohou output; slipzuoqian output; vmin input
function [slipyuohou,slipyouqian,slipzuohou,slipzuoqian] = fcn(vyouhou,vyouqian,vzouhou,vzuoqian,v,vmin)

    v1=vmin;
if v<0.1
    v1 = vmin;
else
    v1 = v;
end
slipyuohou= (vyouhou - v1) / vyouhou;
slipzuohou= (vzouhou - v1) / vzouhou;
slipyouqian= (vyouqian - v1) / vyouqian;
slipzuoqian= (vzuoqian - v1) / vzuoqian;
end

== matlab function finalcode/Subsystem/run/kalman_filter2 ==
  data: a_k_1 input; y output; v_k_1 input; v_k input; V_MIN input; model input
function y = fcn(a_k_1,v_k_1,v_k,V_MIN, model)
A=1;
H=1;
% x_real=v_k_1+0.02*a_k_1;%首先给出一个相应的估计值
% z=0;
% w=0;
% v=0;
% %%噪声信号
%     w=1*randn;
%     v=1*randn;
% %%状态方程
%     x_real=A*v_k_1+0.02*a_k_1+w;
% %%观测方程
%     z=H*x_real+v;
% persistent xhat;
%      % 初始化状态变量
%     if isempty(xhat)
%         xhat = V_MIN;
%     end

    z=H*v_k;
%%kalman_filter  根据上述得观测值来不断更新  
xhat=v_k;
xhat=v_k_1+0.02*a_k_1;%先验估计
Q=1;
R=0.01;
Pk=1;
Pk_bar=0;%先验协方差

    xhat_=v_k_1+0.02*a_k_1;%先验估计
    Pk_bar=A*Pk*A'+Q;
    Kk=Pk_bar*H'/(H*Pk_bar*H'+R);
    xhat= xhat_+ Kk*(z-H* xhat_);%最优估计值
    Pk=(1-Kk*H)*Pk_bar;
if v_k<0.1||model==0||model==9
    y=V_MIN;%即转轮时不使用惯导信息
elseif abs(xhat-v_k)>0.5
    y=v_k;
else
    y = xhat;
end
end

== matlab function finalcode/Subsystem/run/analog_input/无人意图转译/无人/Subsystem1/进esc控制策略/MATLAB Function ==
  data: u input; y output; v input; vd input
function y = fcn(u,v,vd)
persistent vv
if isempty(vv)
    vv=0;
end
if v-vd>0.1*v
    y=vv
else
    y=u;
end
vv=y;

== matlab function finalcode/Subsystem/run/analog_input/MATLAB Function6 ==
  data: model input; y output
function y = fcn(model)
if model~=0||model~=10
    y = 1;
else
    y=0;
end

== matlab function finalcode/Subsystem/run/analog_input/有人/Subsystem1/normal ==
  data: v input; T output
function T = fcn(v)
%#codegen
if v<6000*1.88e-3
    T=2100;
elseif v>11000*1.88e-3
    T=800;
else
    T=1100;
end

== matlab function finalcode/Subsystem/run/analog_input/有人/功率限制/MATLAB Function ==
  data: u1 input; y output; u2 input; u3 input; u4 input
function y = fcn(u1,u2,u3,u4)
sum=(u1+u2+u3+u4)/200;
if sum>75
   a=75/sum;
else
    a=1;
end
y = a;

== matlab function finalcode/Subsystem/run/analog_input/有人/扭矩分配/Enabled Subsystem/LQR差速 ==
  data: yaw_error input; M output; yaw_rate input; J input
% function M = carLQRControl(yaw_error, yaw_rate,J)
%     % 赛车LQR控制器参数
%     Q = diag([1, 1]); % 状态误差权重矩阵
%     R = 0.1; % 控制输入权重
%     
%     % 定义车辆模型参数
%     % J转动惯量
%     
%     % 设计LQR增益矩阵 K
%     A = [0, 1; 0, 0];%输入为期望与实际横摆力矩差值和横摆角速度
%     B = [0; J];
%     K = lqr(A, B, Q, R);
%     
%     % 计算横摆力矩控制输入
%     M = -K* [yaw_error; yaw_rate];
function M = carLQRControl(yaw_error, yaw_rate,J)
    % 赛车LQR控制器参数
    Q = diag([1, 1]); % 状态误差权重矩阵
    R = 0.1; % 控制输入权重
    
    % 设计LQR增益矩阵 K
    A = [0, 1; 0, 0]; % 输入为期望与实际横摆力矩差值和横摆角速度
    B = [0; J];
    
    % 使用迭代法求解代数Riccati方程，计算LQR增益矩阵 K
    max_iterations = 20;
    tolerance = 1e-2;
    P = eye(size(A));
%     for i = 1:max_iterations
%         P_new = Q + A' * P * A - A' * P * B * (R + B' * P * B)^(-1) * B' * P * A;
%         if max(abs(P_new - P), [], 'all') < tolerance
%             P = P_new;
%             break;
%         end
%         P = P_new;
%   K = (R + B' * P * B)^(-1) * B' * P * A;
%     end
     % 计算LQR增益矩阵 

 
   for k = 1:max_iterations
        F = inv(R+B'*P*B)*B'*P*A;
        P_new = (A-B*F)'*P*(A-B*F)+(F)'*R*(F)+Q;
        if max(abs(P_new - P), [], 'all') < tolerance
             P= P_new;
             F = inv(R+B'*P*B)*B'*P*A;
            break;
        end
        P= P_new;
    end
    F_N=F; 
   
    % 计算横摆力矩控制输入
    M = -F_N * [yaw_error; yaw_rate];

end

== matlab function finalcode/Subsystem/run/analog_input/有人/扭矩分配/Enabled Subsystem/MATLAB Function1 ==
  data: w_z input; az output
function az = fcn(w_z)
 % 状态变量
    persistent derivative previous_w_z i
    
    % 初始化状态变量
    if isempty(derivative)
        derivative = 0;
        previous_w_z=0;
        i=0;
    end
derivative = (w_z - previous_w_z)/0.02;
 % 保存上一次数值用于下次计算
    previous_w_z= w_z;
     i=i+1;
az = derivative;
end

== matlab function finalcode/Subsystem/run/analog_input/有人/扭矩分配/Enabled Subsystem/MATLAB Function2 ==
  data: angle input; y output; M input
 function y = fcn(angle,M)
if angle>10||angle<-10%4650000,4870000,4741002
    y=M;
else
    y = 0;
end

== matlab function finalcode/Subsystem/run/analog_input/有人/扭矩分配/Enabled Subsystem/kalman_filter ==
  data: a_k_1 input; y output; w_k_1 input; w_k input; w_z2 input
function y = fcn(a_k_1,w_k_1,w_k,w_z2)
A=1;
H=1;
persistent integral  Kk
  if isempty(integral)
        integral = 0;
         xhat = w_k_1;
    end
% x_real=v_k_1+0.02*a_k_1;%首先给出一个相应的估计值
% z=0;
% w=0;
% v=0;
% %%噪声信号
%     w=1*randn;
%     v=1*randn;
% %%状态方程
%     x_real=A*v_k_1+0.02*a_k_1+w;
% %%观测方程
%     z=H*x_real+v;
% persistent xhat;
%      % 初始化状态变量
%     if isempty(xhat)
%         xhat = V_MIN;
%     end

    z=H*w_k;
%%kalman_filter  根据上述得观测值来不断更新  
xhat=w_k;
xhat=w_k_1+0.02*a_k_1;%先验估计
Q=1;
R=0.01;
Pk=1;
Pk_bar=0;%先验协方差

    xhat_=w_k_1+0.02*a_k_1;%先验估计
    Pk_bar=A*Pk*A'+Q;
    Kk=Pk_bar*H'/(H*Pk_bar*H'+R);
    xhat= xhat_+ Kk*(z-H* xhat_);%最优估计值
    Pk=(1-Kk*H)*Pk_bar;
if w_k<0.1
    y=w_z2;%即转轮时不使用惯导信息
elseif abs(xhat-w_k)>0.5
    y=w_k;
else
    y = xhat;
end
end

== matlab function finalcode/Subsystem/run/analog_input/有人/扭矩分配/Enabled Subsystem/期望横摆力矩计算 ==
  data: delta input; Mz output; Vx input; ax input
function Mz = calculateYawMoment(delta,  Vx, ax)
    % 输入参数：
    % delta: 前轮转角 (rad)
    % Vx: 车辆速度 (m/s)
    % ax: 侧向加速度 (m/s^2)
    m=210;%: 车辆质量 (kg)
     lf=0.765;%: 前轴到重心的距离 (m)
     lr=0.765;%: 后轴到重心的距离 (m)
    
    % 轮胎侧向力估计，这里使用一个简化的线性模型
    Fy = ax * (lr * m * 9.81) / (lf + lr);
    delta=delta*pi/180
    % 计算期望的横摆力矩
    Mz = lf * Fy * cos(delta);
end

== matlab function finalcode/Subsystem/Tx/TX控制器/速度/189左后/MATLAB Function6 ==
  data: v input; T output; a input
function T = fcn(v,a)
% if a>5
%     y = u;
% elseif a>3&&a<5
%     y=1200;
% else
%     y=800;
% end

if v<6000*1.88e-3
    T=2100;
elseif v>11000*1.88e-3
    T=800;
else
    T=1100;
end

== matlab function finalcode/Subsystem/run/analog_input/有人/扭矩分配/Enabled Subsystem/横摆角速度 ==
  data: ay input; wz1 output; wz2 output; vx input; vfr input; vfl input; vrl input; vrr input; Bf input; alpha input; k input
function [wz1,wz2]= fcn(ay,vx,vfr,vfl,vrl,vrr,Bf,alpha,k)
wz1=ay/vx;
wz2_1=(vfr-vfl)/Bf*cos(alpha);
wz2_2=(vrr-vrl)/Bf;
wz2=wz2_1*k+wz2_2*(1-k);
% lrr为轮距

== matlab function finalcode/Subsystem/run/analog_input/有人/扭矩分配/MATLAB Function ==
  data: M input; M_qian output; ax input; M_hou output; k input
function [M_qian,M_hou]= fcn(M,ax,k)

dot_M1=k*ax;
if dot_M1>200
    dot_M=200;
else
    dot_M=dot_M1;
end
M_qian = 0.6* M-dot_M;
M_hou  = 0.4* M+dot_M;

== matlab function finalcode/Subsystem/run/analog_input/有人/扭矩分配/MATLAB Function3 ==
  data: M_qian input; M_hou input; youhou output; M input; youqian output; zuohou output; zuoqian output
function [youhou,youqian,zuohou,zuoqian] = fcn(M_qian,M_hou,M)
% U=4*u;
r=0.2032;%轮半径
B1=1.18;%左右轮距
B2=1.16;
youqian=M*r/(2*B2)+M_qian;
zuoqian=-M*r/(2*B1)+M_qian;
youhou=M*r/(2*B2)+M_hou;
zuohou=-M*r/(2*B1)+M_hou;
end

== matlab function finalcode/Subsystem/run/analog_input/有人/限滑/Enabled Subsystem/MATLAB Function ==
  data: v input; v_history input; J input; M output; M_history input; minus output
function [M,minus]= fcn(v,v_history,J,M_history)

% 状态变量
    persistent   u
    
    % 初始化状态变量
    if isempty(minus)
         minus = 0;
        M=M_history;
    end
    
    minus = v- v_history;
    
    Q = 1; % 状态误差权重矩阵
    R = 0.1; % 控制输入权重
    A = 1; 
    B = 0.02*M/J;
    
    max_iterations = 20;
    tolerance = 1e-2;
    P = eye(size(A));
    for k = 1:max_iterations
        F = inv(R+B'*P*B)*B'*P*A;
        P_new = (A-B*F)'*P*(A-B*F)+(F)'*R*(F)+Q;
        if max(abs(P_new - P), [], 'all') < tolerance
             P= P_new;
             F = (R+B'*P*B)\B'*P*A;
            break;
        end
        P= P_new;
    end
    F_N=F; 
    M = -F_N * v;
    u=M;
    

   y = M;

end

== matlab function finalcode/Subsystem/run/analog_input/有人/限滑/Enabled Subsystem/MATLAB Function1 ==
  data: u1 input; y output; u2 input
function y = fcn(u1,u2)
if slip_ratio >0.5&& minus>1000
y = u1;
elseif slip_ratio <-0.5&& minus>1000
y = u1;
else
    y=u2;
end

== matlab function finalcode/Subsystem/run/analog_input/有人/限滑/Enabled Subsystem/pid限滑 ==
  data: slip input; M output; slip_ratio_limit input; u input
function M  = carPIDWithSlipControl(slip, slip_ratio_limit,u)
    % 赛车PID控制器参数
    kp = 0.2;
    ki = 0.1;
    kd = 0.01;
    
    % 状态变量
    persistent integral previous_error i
    
    % 初始化状态变量
    if isempty(integral)
        integral = 0;
        previous_error = 0;
        i=0;
    end
    
    % PID控制器计算
    error = 0.2 - slip;
    integral = integral + error*0.02;
    derivative = (error - previous_error)/0.02;
    
   k = kp * error + ki * integral + kd * derivative;
     output = u+k*u;
    if output>2000
       output=2000;
    else
        output=u;
    end
     if slip > slip_ratio_limit
        
        M = 0;
    % 根据滑移率限制输出
     else
        M=output;
     end
    % 保存上一个误差用于下次计算
    previous_error = error;

    i=i+1;
end

== matlab function finalcode/Subsystem/run/analog_input/有人/限滑/Enabled Subsystem/pid限滑1 ==
  data: slip input; M output; slip_ratio_limit input; u input
function M  = carPIDWithSlipControl(slip, slip_ratio_limit,u)
    % 赛车PID控制器参数
    kp = 0.2;
    ki = 0.1;
    kd = 0.01;
    
    % 状态变量
    persistent integral previous_error i
    
    % 初始化状态变量
    if isempty(integral)
        integral = 0;
        previous_error = 0;
        i=0;
    end
    
    % PID控制器计算
    error = 0.2 - slip;
    integral = integral + error*0.02;
    derivative = (error - previous_error)/0.02;
    
   k = kp * error + ki * integral + kd * derivative;
     output = u+k*u;
    if output>2000
       output=2000;
    else
        output=u;
    end
     if slip > slip_ratio_limit
        
        M = 0;
    % 根据滑移率限制输出
     else
        M=output;
     end
    % 保存上一个误差用于下次计算
    previous_error = error;

    i=i+1;
end

== matlab function finalcode/Subsystem/Tx/TX控制器/速度/185右前/MATLAB Function2 ==
  data: enable input; enable_1 input; T input; TargetVelocity output; AMK_TorqueLimitPositive output; enable output; errorreset output; blnverteron output; CAN_dbcon output; v input
function [TargetVelocity,AMK_TorqueLimitPositive,enable,errorreset,blnverteron,CAN_dbcon]= fcn(enable,enable_1,T,v)
if (enable_1==0)
    TargetVelocity=0;
    enable=0;
    errorreset=1;
    blnverteron=0;
    CAN_dbcon=0;
    AMK_TorqueLimitPositive=0;
elseif (enable==0 && enable_1==1)
    TargetVelocity=2000;
    enable=1;
    errorreset=0;
    blnverteron=1;
    CAN_dbcon=1;
    AMK_TorqueLimitPositive=0;
elseif (enable==1 && enable_1==1)
    TargetVelocity=2000;
    enable=1;
    errorreset=0;
    blnverteron=1;
    CAN_dbcon=1;
    AMK_TorqueLimitPositive=T;
else
    TargetVelocity=0;
    enable=0;
    errorreset=1;
    blnverteron=0;
    CAN_dbcon=0;
    AMK_TorqueLimitPositive=0;
end

end

== matlab function finalcode/Subsystem/run/analog_input/有人/限滑/Enabled Subsystem/pid限滑2 ==
  data: slip input; M output; slip_ratio_limit input; u input
function M  = carPIDWithSlipControl(slip, slip_ratio_limit,u)
    % 赛车PID控制器参数
    kp = 0.2;
    ki = 0.1;
    kd = 0.01;
    
    % 状态变量
    persistent integral previous_error i
    
    % 初始化状态变量
    if isempty(integral)
        integral = 0;
        previous_error = 0;
        i=0;
    end
    
    % PID控制器计算
    error = 0.2 - slip;
    integral = integral + error*0.02;
    derivative = (error - previous_error)/0.02;
    
   k = kp * error + ki * integral + kd * derivative;
     output = u+k*u;
    if output>2000
       output=2000;
    else
        output=u;
    end
     if slip > slip_ratio_limit
        
        M = 0;
    % 根据滑移率限制输出
     else
        M=output;
     end
    % 保存上一个误差用于下次计算
    previous_error = error;

    i=i+1;
end

== matlab function finalcode/Subsystem/run/analog_input/有人/限滑/Enabled Subsystem/pid限滑3 ==
  data: slip input; M output; slip_ratio_limit input; u input
function M  = carPIDWithSlipControl(slip, slip_ratio_limit,u)
    % 赛车PID控制器参数
    kp = 0.2;
    ki = 0.1;
    kd = 0.01;
    
    % 状态变量
    persistent integral previous_error i
    
    % 初始化状态变量
    if isempty(integral)
        integral = 0;
        previous_error = 0;
        i=0;
    end
    
    % PID控制器计算
    error = 0.2 - slip;
    integral = integral + error*0.02;
    derivative = (error - previous_error)/0.02;
    
   k = kp * error + ki * integral + kd * derivative;
     output = u+k*u;
    if output>2000
       output=2000;
    else
        output=u;
    end
     if slip > slip_ratio_limit
        
        M = 0;
    % 根据滑移率限制输出
     else
        M=output;
     end
    % 保存上一个误差用于下次计算
    previous_error = error;

    i=i+1;
end

== matlab function finalcode/Subsystem/run/analog_input/有人/限滑/MATLAB Function ==
  data: u input; y output
function y = fcn(u)
% if -5<u&&u<=5
%     y=0;
% else
%     y=1;
y=0;
end

== matlab function finalcode/Subsystem/Rx/shucai—receive/Subsystem1/Subsystem/MATLAB Function ==
  data: x input; ax output; y input; z input; ay output; az output
function [ax,ay,az]= fcn(x,y,z)

ax = x/32768*16*9.7988;
ay = y/32768*16*9.7988;
az = z/32768*16*9.7988;
